simulink library "HeatExchanger"  (Simulink 8.2)
settings: Solver=ode45  StartTime=0.0  StopTime=10.0  RelTol=1e-3
libraries: carnot x2
settings Model: Creator=lena.frank  LastModifiedBy=drhf

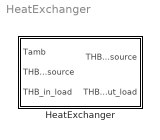
== system HeatExchanger ==
  HeatExchanger : Subsystem  mask(heat exchanger){flowtype=1, ua0=2000, uahot=[0.04 0], uacold=[0.04 0], ualoss=3, cap=10e3, linh=20, quah=10, linc=20, quac=10, t0=20}
      mask prompts: flowtype "type of flow (0 = parallel, 0.5 = cross, 1 = counter)"; ua0 "constant heat transfer ua0 [W/K]"; uahot "[mdot_nom_hot [kg/s] (>0) ,  ua_exp_hot (>=0)]"; uacold "[mdot_nom_cold [kg/s] (>0) ,  ua_exp_cold (>=0)]"; ualoss "heat losses to ambient [W/K]"; cap "capacity [J/K]"; linh "Source: pressure drop linear in massflow [Pa*s/kg]"; quah "Source: pressure drop quadratic in massflow [Pa*s²/kg²]"; linc "Load: pressure drop linear in massflow [Pa*s/kg]"; quac "Load: pressure drop quadratic in massflow [Pa*s²/kg²]"; t0 "initial temperature [degree centigrade]"
      mask help:
      | Calculates the output THV of the hot and cold fluid of a heat exchanger.
      | The heat transfer is:
      | ua = ua0 * ( (mdot_hot/mdot_nom_hot)^ua_exp_hot
      |      + (mdot_cold/mdot_nom_cold)^ua_exp_cold )/2
      mask init:
      | flowtype = max(0, min(flowtype, 1));
      | linh = max(linh,0);
      | linc = max(linc,0);
      | quah = max(quah,0);
      | quac = max(quac,0);
      | uahot(1) = max(uahot(1), 1e-4);
      | uahot(2) = max(uahot(2), 0);
      | uacold(1) = max(uacold(1), 1e-4);
      | uacold(2) = max(uacold(2), 0);
      | cap = max(cap, 0.01);
      mask Help: web(fullfile(path_carnot('help'),'HeatExchanger.html'),'-helpbrowser')
      mask Display:
      | plot(-10,20,115,100,[40,70,70,40,40],[40 40 70 70 40],[55 55 62 48 55 55],[25 40 55 55 70 85],[30 40],[55 55],[70 80],[55 55])
      | port_label('input',1,'Ta')
      | port_label('input',2,'THBpri')
      | port_label('input',3,'THBsec')
      | port_label('output',1,'THBpri')
      | port_label('output',2,'THBsec')

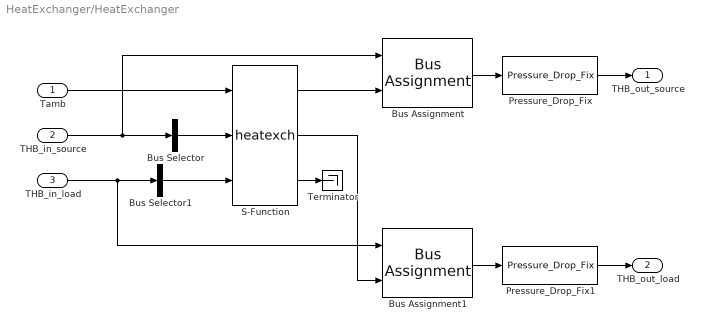
== system HeatExchanger/HeatExchanger ==
  Tamb : Inport
  THB_in_source : Inport  Port=2
  THB_in_load : Inport  Port=3
  Bus Assignment : BusAssignment  AssignedSignals=Temperature
  Bus Assignment1 : BusAssignment  AssignedSignals=Temperature
  Bus Selector : BusSelector  OutputSignals=Temperature,MassFlow,Pressure,FluidType,FluidMix  OutputAsBus=on
  Bus Selector1 : BusSelector  OutputSignals=Temperature,MassFlow,Pressure,FluidType,FluidMix  OutputAsBus=on
  Pressure_Drop_Fix : carnot/Basic/Pressure_Drop/Pressure_Drop_Fix  con=0  lin=linh  qua=quah
  Pressure_Drop_Fix1 : carnot/Basic/Pressure_Drop/Pressure_Drop_Fix  con=0  lin=linc  qua=quac
  S-Function : S-Function  FunctionName=heatexch  Parameters=flowtype, ua0, uahot(1), uahot(2), uacold(1), uacold(2), ualoss, cap, t0  EnableBusSupport=off
  Terminator : Terminator
  THB_out_source : Outport
  THB_out_load : Outport  Port=2
  wires:
  Tamb/1 -> S-Function/1
  Bus Selector/1 -> S-Function/2
  S-Function/3 -> Terminator/1
  THB_in_source/1 -> Bus Selector/1, Bus Assignment/1
  THB_in_load/1 -> Bus Selector1/1, Bus Assignment1/1
  Bus Selector1/1 -> S-Function/3
  S-Function/1 -> Bus Assignment/2
  Bus Assignment/1 -> Pressure_Drop_Fix/1
  S-Function/2 -> Bus Assignment1/2
  Bus Assignment1/1 -> Pressure_Drop_Fix1/1
  Pressure_Drop_Fix/1 -> THB_out_source/1
  Pressure_Drop_Fix1/1 -> THB_out_load/1
